simulink model "MFunction1"  (R2017b)
settings: Solver=FixedStepAuto  StartTime=0.0  StopTime=10.0  FixedStep=1.000000  RelTol=1e-3
settings Model: Creator=hbourbou  LastModifiedBy=hbourbou

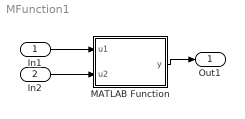
== system MFunction1 ==
  In1 : Inport
  In2 : Inport  Port=2
  MATLAB Function : MATLAB Function  TreatAsAtomicUnit=on
  Out1 : Outport
  wires:
  In1/1 -> MATLAB Function/1(u1)
  MATLAB Function/1(y) -> Out1/1
  In2/1 -> MATLAB Function/2(u2)

== matlab function MFunction1/MATLAB Function ==
  data: u1 input; y output; u2 input
function y = fcn(u1, u2)
y = and(u1, u2);
